simulink model "arduino_robotics_motors_gettingstarted"  (R2023b)
settings: Solver=ode3  StartTime=0.0  StopTime=inf  RelTol=1e-3  EnableMultiTasking=on
libraries: arduinolib x4, simulink x2
settings Model: FPTRunName=Active  ExtModeTrigDuration=2  Creator=The MathWorks, Inc.  LastModifiedBy=maxju
settings SolverCC: AlgebraicLoopSolver=TrustRegion
settings DataIOCC: LimitDataPoints=on  ReturnWorkspaceOutputs=off
settings OptimizationCC: ReuseModelBlockBuffer=off  ExpressionDepthLimit=2147483647  LifeSpan=Inf  MaxStackSize=64
settings DebuggingCC: MergeDetectMultiDrivingBlocksExec=none  FcnCallInpInsideContextMsg=warning  UnconnectedInputMsg=warning  UnconnectedOutputMsg=warning  UnconnectedLineMsg=warning  AllowSymbolicDim=off  StateNameClashWarn=warning  SFUnexpectedBacktrackingDiag=warning  SFNoUnconditionalDefaultTransitionDiag=warning  SFExecutionAtInitializationDiag=none  ArithmeticOperatorsInVariantConditions=warning
settings HardwareCC: ProdBitPerInt=16  ProdBitPerPointer=16  ProdBitPerSizeT=16  ProdBitPerPtrDiffT=16  ProdLargestAtomicFloat=None  ProdWordSize=8  ProdHWDeviceType=Atmel->AVR  UseEmbeddedCoderFeatures=off  UseSimulinkCoderFeatures=off
settings ModelReferenceCC: EnableRefExpFcnMdlSchedulingChecks=on  PropagateSignalLabelsOutOfModel=off
settings SFSimCC: SimUseLocalCustomCode=off  MATLABDynamicMemAlloc=off
settings RTWCC: Description=Embedded Coder  SystemTargetFile=ert.tlc  HardwareBoard=Arduino Uno  TemplateMakefile=ert_default_tmf  GenerateReport=on  RTWVerbose=off  RTWUseLocalCustomCode=off  Toolchain=Arduino AVR  BuildConfiguration=Faster Runs  LaunchReport=on  DLArmComputeVersion=19.05
settings CodeAppCC: ForceParamTrailComments=on  OperatorAnnotations=on  StateflowObjectComments=on  MATLABSourceComments=on
settings ERTTargetCC: MultiwordLength=2048  ERTCustomFileBanners=off  SupportContinuousTime=on  SupportNonInlinedSFcns=on  RemoveResetFunc=off  SupportVariableSizeSignals=on  ModelStepFunctionPrototypeControlCompliant=off  ExtModeTransport=3  ExtModeStaticAlloc=on  ExtModeAutomaticAllocSize=off  ExtModeStaticAllocSize=250  ExtModeMexFile=ext_xcp  ExtModeIntrfLevel=Level2 - Open
settings ConfigComp: CovMetricSettings=dw  CovSaveCumulativeToWorkspaceVar=on  CovSaveSingleToWorkspaceVar=on  CovExternalEMLEnable=off  CovSFcnEnable=off

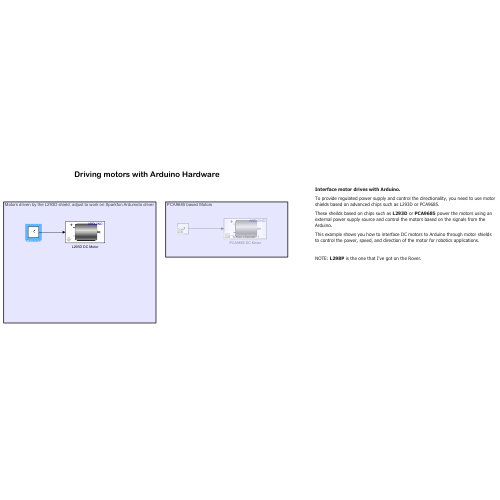
[thumbnail: Simulink's stored preview of the top-level diagram]
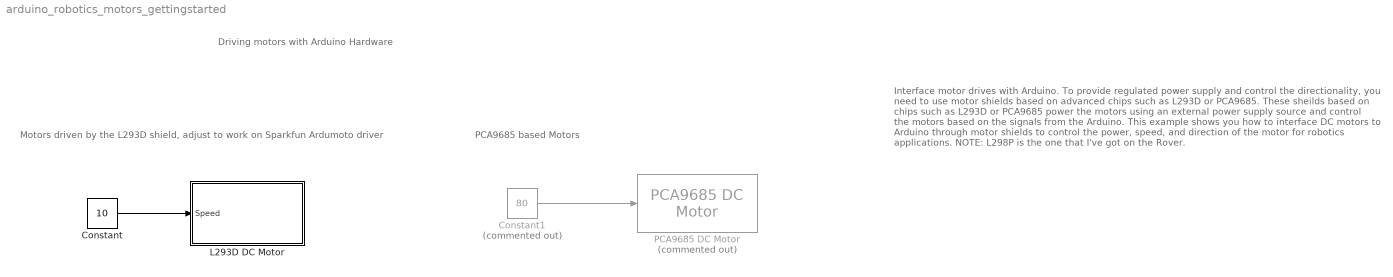
== system arduino_robotics_motors_gettingstarted ==
  note: Interface motor drives with Arduino.
      | To provide regulated power supply and control the directionality, you need to use motor shields based on advanced chips such as L293D or PCA9685.
      | These sheilds based on chips such as L293D or PCA9685 power the motors using an external power supply source and control the motors based on the signals from the Arduino.
      | This example shows you how to interface DC motors to Arduino through motor shields to control the power, speed, and direction of the motor for robotics applications.
      |
      | NOTE: L298P is the one that I've got on the Rover.
  note: Motors driven by the L293D shield, adjust to work on Sparkfun Ardumoto driver
  note: Driving motors with Arduino Hardware
  note: PCA9685 based Motors
  Constant : Constant  Value=10  SampleTime=0.1
  Constant1 : Constant  Commented=on  Value=80  SampleTime=0.1
  L293D DC Motor : Subsystem  AncestorBlock=arduinolib/L293D DC Motor  mask{EnablePin=5, InputAPin=3, InputBPin=11}
      mask prompts: EnablePin "arduino:blockmask:L293DDCMotorEnablePinProp"; InputAPin "arduino:blockmask:L293DDCMotorInputAPinProp"; InputBPin "arduino:blockmask:L293DDCMotorInputBPinProp"
      mask Help: eval('codertarget.internal.helpView(''arduinoert'', ''arduinoL293DDCMotor'')')
      mask TypeOptions EnablePin: PWMSelection/pinNumber
      mask TypeOptions InputAPin: Digital Output/pinNumber
      mask TypeOptions InputBPin: Digital Output1/pinNumber
      mask DialogControl DescGroupVar Prompt: L293D DC Motor
      mask DialogControl DescTextVar Prompt: arduino:blockmask:L293DDCMotorBlockDescription
      mask DialogControl EnablePin Prompt: Enable pin
      mask DialogControl InputAPin Prompt: Input A pin
      mask DialogControl InputBPin Prompt: Input B pin
      mask Display:
      | color('white');
      | plot([100,100,100,100]*1,[100,100,100,100]*1);
      | plot([100,100,100,100]*0,[100,100,100,100]*0);
      | color('black');
      | sppkgroot = strrep(codertarget.arduinobase.internal.getBaseSpPkgRootDir(),'\','/');
      | image(fullfile(sppkgroot,'resources','dcmotor.png'),'center')
      | color('blue');
      | text(99, 92, '\fontsize{9}ARDUINO ','texmode','on','horizontalAlignment', 'right');
      | color('black');
  PCA9685 DC Motor : arduinolib/PCA9685 DC Motor  Commented=on  PCA9685Address=0x60  PWMFrequency=1200  MotorChannel=1
  wires:
  Constant/1 -> L293D DC Motor/1(Speed)
  Constant1/1 -> PCA9685 DC Motor/1

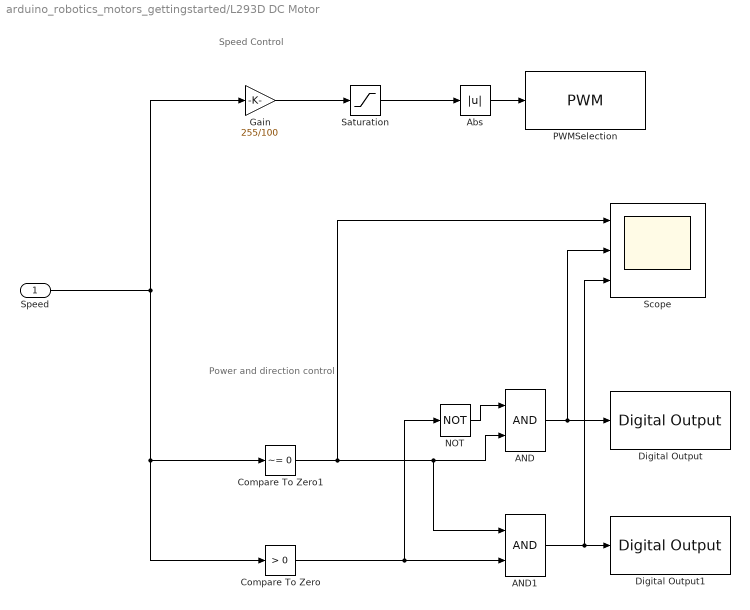
== system arduino_robotics_motors_gettingstarted/L293D DC Motor ==
  note: Power and direction control
  note: Speed Control
  Speed : Inport
  AND : Logic  IconShape=distinctive  AllPortsSameDT=off  OutDataTypeStr=boolean
  AND1 : Logic  IconShape=distinctive  AllPortsSameDT=off  OutDataTypeStr=boolean
  Abs : Abs  SaturateOnIntegerOverflow=off
  Compare To Zero : simulink/Logic and Bit Operations/Compare To Zero  relop=>  OutDataTypeStr=boolean
  Compare To Zero1 : simulink/Logic and Bit Operations/Compare To Zero  relop=~=  OutDataTypeStr=boolean
  Digital Output : arduinolib/Digital Output  pinNumber=InputAPin  Direction=output  blockPlatform=arduino
      settings: LibrarySourceBlock=arduinolib/L293D DC Motor/Digital Output
  Digital Output1 : arduinolib/Digital Output  pinNumber=InputBPin  Direction=output  blockPlatform=arduino
      settings: LibrarySourceBlock=arduinolib/L293D DC Motor/Digital Output1
  Gain : Gain  Gain=255/100
  NOT : Logic  Operator=NOT  IconShape=distinctive  AllPortsSameDT=off  OutDataTypeStr=boolean
  PWMSelection : arduinolib/PWM  pinNumber=EnablePin  frequencyType=Default  desiredFrequency=490.2  achievableFrequency=490.2
      settings: LibrarySourceBlock=arduinolib/L293D DC Motor/PWMSelection
  Saturation : Saturate  UpperLimit=255  LowerLimit=-255
  Scope : Scope  NumInputPorts=3
  wires:
  Saturation/1 -> Abs/1
  Gain/1 -> Saturation/1
  Speed/1 -> Compare To Zero/1, Compare To Zero1/1, Gain/1
  Compare To Zero/1 -> NOT/1, AND1/2
  AND1/1 -> Scope/3, Digital Output1/1
  Compare To Zero1/1 -> Scope/1, AND1/1, AND/2
  AND/1 -> Scope/2, Digital Output/1
  NOT/1 -> AND/1
  Abs/1 -> PWMSelection/1
